simulink model "ddr"  (R2020b)
settings: Solver=VariableStepAuto  StartTime=0.0  StopTime=10.0  RelTol=1e-3
model workspace (MAT data in the model file):
  Var = 2
  Var1 = 6
  Var2 = 8
  Var3 = 0
values from neighbouring files (symbols this model uses):
  A = 2.0    [Ddr2.sldd]    (also in Untitled2.m = 10)
  B = 2.0    [Ddr2.sldd]
  C = 3.0    [Ddr2.sldd]
settings Model: DataDictionary=Ddr2.sldd  Creator=sai  LastModifiedBy=sai

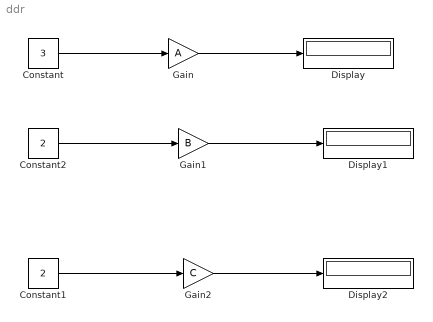
== system ddr ==
  Constant : Constant  Value=3
  Constant1 : Constant  Value=2
  Constant2 : Constant  Value=2
  Display : Display
  Display1 : Display
  Display2 : Display
  Gain : Gain  Gain=A
  Gain1 : Gain  Gain=B
  Gain2 : Gain  Gain=C
  wires:
  Gain2/1 -> Display2/1
  Gain1/1 -> Display1/1
  Gain/1 -> Display/1
  Constant/1 -> Gain/1
  Constant2/1 -> Gain1/1
  Constant1/1 -> Gain2/1
